simulink model "FOC"  (R2025a)
settings: Solver=VariableStepAuto  StartTime=0.0  StopTime=15  MaxStep=1e-4  RelTol=1e-3
undefined symbols (not defined in the file or in its folder): P
settings Model: Creator=20374  LastModifiedBy=20374

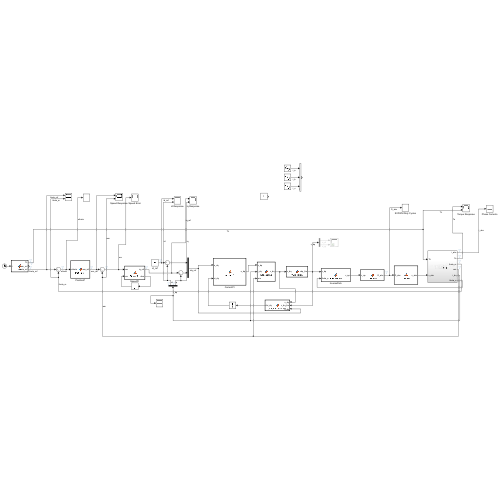
[thumbnail: Simulink's stored preview of the top-level diagram]
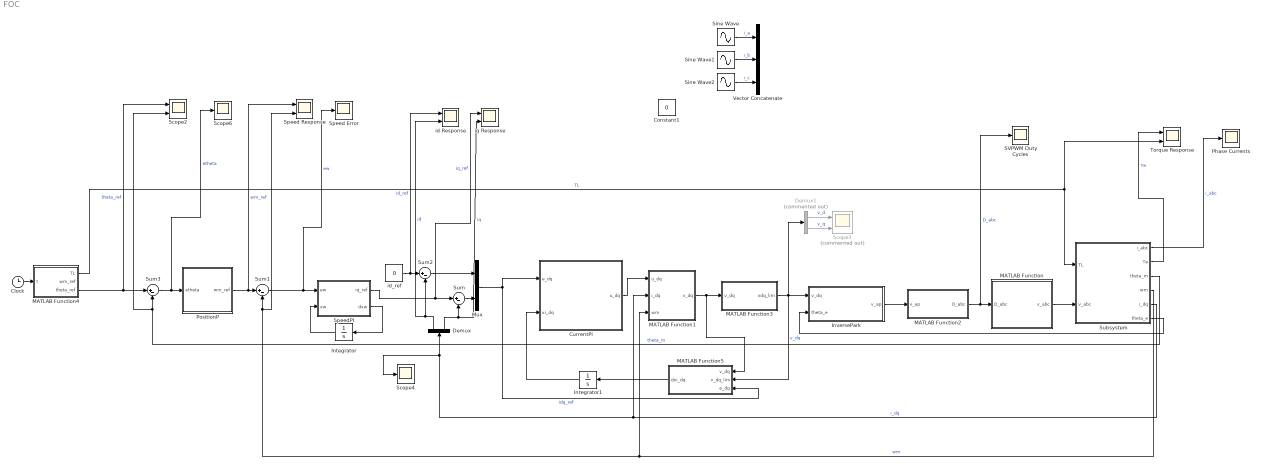
== system FOC ==
  Clock : Clock
  Constant1 : Constant  Value=0
  CurrentPI : MATLAB Function  TreatAsAtomicUnit=on
  Demux : Demux  Outputs=2
  Demux1 : Demux  Commented=on  Outputs=2
  Integrator : Integrator
  Integrator1 : Integrator
  InversePark : MATLAB Function  TreatAsAtomicUnit=on
  MATLAB Function : MATLAB Function  TreatAsAtomicUnit=on
  MATLAB Function1 : MATLAB Function  TreatAsAtomicUnit=on
  MATLAB Function2 : MATLAB Function  TreatAsAtomicUnit=on
  MATLAB Function3 : MATLAB Function  TreatAsAtomicUnit=on
  MATLAB Function4 : MATLAB Function  TreatAsAtomicUnit=on
  MATLAB Function5 : MATLAB Function  TreatAsAtomicUnit=on
  Mux : Mux  Inputs=2
  Phase Currents : Scope
      settings: DataLoggingVariableName=ScopeData9
  PositionP : MATLAB Function  TreatAsAtomicUnit=on
  SVPWM Duty Cycles : Scope
      settings: DataLoggingVariableName=ScopeData10
  Scope2 : Scope  NumInputPorts=2
      settings: ActiveDisplayYMinimum=-0.94255582944126726  ActiveDisplayYMaximum=16.800284873719775  DataLoggingVariableName=ScopeData2
  Scope3 : Scope  Commented=on  NumInputPorts=2
      settings: ActiveDisplayYMinimum=-185.69935334057905  ActiveDisplayYMaximum=341.38341103207864  DataLoggingVariableName=ScopeData3
  Scope4 : Scope
      settings: ActiveDisplayYMinimum=-1.2499772986958553  ActiveDisplayYMaximum=11.249795688208886  DataLoggingVariableName=ScopeData4
  Scope6 : Scope
      settings: ActiveDisplayYMinimum=-1.1047635267751033  ActiveDisplayYMaximum=7.10408082072833  DataLoggingVariableName=ScopeData7
  Sine Wave : Sin  Frequency=20*pi  SampleTime=0
  Sine Wave1 : Sin  Phase=2*pi/3  SampleTime=0
  Sine Wave2 : Sin  Phase=-2*pi/3  SampleTime=0
  Speed Error : Scope
      settings: ActiveDisplayYMinimum=-30.007135590035606  ActiveDisplayYMaximum=73.147296256443809  DataLoggingVariableName=ScopeData6
  Speed Response : Scope  NumInputPorts=2
      settings: ActiveDisplayYMinimum=-19.63649397524663  ActiveDisplayYMaximum=176.72844577721969  DataLoggingVariableName=ScopeData8
  SpeedPI : MATLAB Function  TreatAsAtomicUnit=on
  Subsystem : Subsystem
  Sum{,1..3} (4 alike) : Sum  Inputs=|+-
  Torque Response : Scope  NumInputPorts=2
      settings: DataLoggingVariableName=ScopeData5
  Vector Concatenate : Concatenate  NumInputs=3  Mode=Multidimensional array
  id Response : Scope  NumInputPorts=2
      settings: ActiveDisplayYMinimum=-27.477041816535841  ActiveDisplayYMaximum=247.29337634882265
  id_ref : Constant  Value=0
  iq Response : Scope  NumInputPorts=2
      settings: ActiveDisplayYMinimum=-6.574069056505973  ActiveDisplayYMaximum=11.841563228500664
  wires:
  Sine Wave/1 -> Vector Concatenate/1  "i_a"
  Sine Wave1/1 -> Vector Concatenate/2  "i_b"
  Sine Wave2/1 -> Vector Concatenate/3  "i_c"
  Integrator1/1 -> CurrentPI/2(xi_dq)
  CurrentPI/1(u_dq) -> MATLAB Function1/1(u_dq)
  Subsystem/6(theta_e) -> InversePark/2(theta_e)
  MATLAB Function/1(v_abc) -> Subsystem/2(v_abc)
  MATLAB Function2/1(D_abc) -> SVPWM Duty Cycles/1, MATLAB Function/1(D_abc)  "D_abc"
  InversePark/1(v_ap) -> MATLAB Function2/1(v_ap)
  Subsystem/5(i_dq) -> MATLAB Function1/2(i_dq), Scope4/1, Demux/1  "i_dq"
  Sum1/1 -> Speed Error/1, SpeedPI/1(ew)  "ew"
  Subsystem/4(wm) -> MATLAB Function1/3(wm), Speed Response/2, Sum1/2  "wm"
  MATLAB Function3/1(vdq_lim) -> Demux1/1, MATLAB Function5/2(v_dq_lim), InversePark/1(v_dq)  "v_dq"
  MATLAB Function1/1(v_dq) -> MATLAB Function5/1(v_dq), MATLAB Function3/1(v_dq)
  MATLAB Function4/1(TL) -> Torque Response/2, Subsystem/1(TL)  "TL"
  Clock/1 -> MATLAB Function4/1(t)
  Mux/1 -> CurrentPI/1(e_dq), MATLAB Function5/3(e_dq)  "idq_ref"
  Sum2/1 -> Mux/1
  Sum/1 -> Mux/2
  SpeedPI/1(iq_ref) -> iq Response/1, Sum/1  "iq_ref"
  id_ref/1 -> id Response/1, Sum2/1  "id_ref"
  Demux1/1 -> Scope3/1  "v_d"
  Demux1/2 -> Scope3/2  "v_q"
  Demux/1 -> Sum2/2, id Response/2  "id"
  Demux/2 -> Sum/2, iq Response/2  "iq"
  SpeedPI/2(dxw) -> Integrator/1
  Integrator/1 -> SpeedPI/2(xw)
  MATLAB Function5/1(dxi_dq) -> Integrator1/1
  Subsystem/3(theta_m) -> Scope2/2, Sum3/2  "theta_m"
  MATLAB Function4/3(theta_ref) -> Sum3/1, Scope2/1  "theta_ref"
  Sum3/1 -> Scope6/1, PositionP/1(etheta)  "etheta"
  Subsystem/2(Te) -> Torque Response/1  "Te"
  Subsystem/1(i_abc) -> Phase Currents/1  "i_abc"
  PositionP/1(wm_ref) -> Speed Response/1, Sum1/1  "wm_ref"

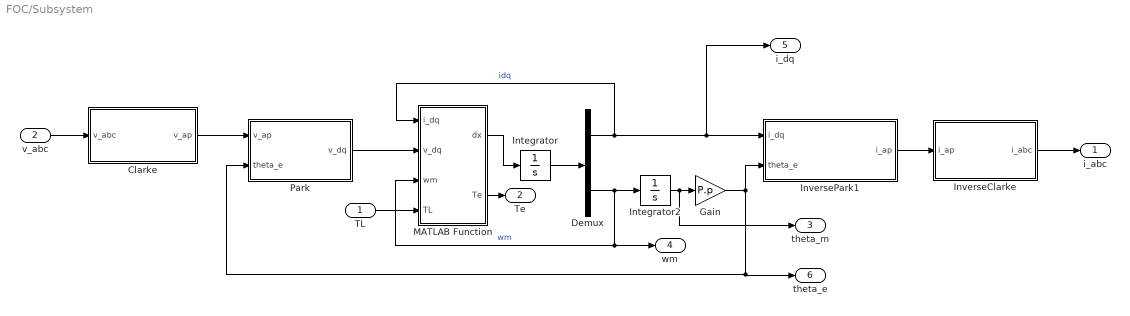
== system FOC/Subsystem ==
  TL : Inport
  v_abc : Inport  Port=2
  Clarke : MATLAB Function  TreatAsAtomicUnit=on
  Demux : Demux  Outputs=[2,1]
  Gain : Gain  Gain=P.p
  Integrator : Integrator  InitialCondition=[0;0;0]
  Integrator2 : Integrator
  InverseClarke : MATLAB Function  TreatAsAtomicUnit=on
  InversePark1 : MATLAB Function  TreatAsAtomicUnit=on
  MATLAB Function : MATLAB Function  TreatAsAtomicUnit=on
  Park : MATLAB Function  TreatAsAtomicUnit=on
  i_abc : Outport
  Te : Outport  Port=2
  theta_m : Outport  Port=3
  wm : Outport  Port=4
  i_dq : Outport  Port=5
  theta_e : Outport  Port=6
  wires:
  InversePark1/1(i_ap) -> InverseClarke/1(i_ap)
  Demux/2 -> wm/1, MATLAB Function/3(wm), Integrator2/1  "wm"
  Demux/1 -> i_dq/1, InversePark1/1(i_dq), MATLAB Function/1(i_dq)  "idq"
  Integrator2/1 -> theta_m/1, Gain/1
  Gain/1 -> theta_e/1, Park/2(theta_e), InversePark1/2(theta_e)
  TL/1 -> MATLAB Function/4(TL)
  Integrator/1 -> Demux/1
  InverseClarke/1(i_abc) -> i_abc/1
  MATLAB Function/1(dx) -> Integrator/1
  Clarke/1(v_ap) -> Park/1(v_ap)
  Park/1(v_dq) -> MATLAB Function/2(v_dq)
  v_abc/1 -> Clarke/1(v_abc)
  MATLAB Function/2(Te) -> Te/1

== matlab function FOC/MATLAB Function ==
  data: D_abc input; v_abc output; P parameter
function v_abc = Inverter(D_abc,P)

Da = D_abc(1);
Db = D_abc(2);
Dc = D_abc(3);

Vdc = P.Vdc;

va = Vdc/3 * (2*Da-Db-Dc);
vb = Vdc/3 * (2*Db-Da-Dc);
vc = Vdc/3 * (2*Dc-Da-Db);

v_abc = [va; vb; vc];

end

== matlab function FOC/MATLAB Function2 ==
  data: v_ap input; D_abc output; P parameter
function D_abc = SVPWM(v_ap,P)

v_alpha = v_ap(1);
v_beta  = v_ap(2);

Vdc = P.Vdc;
Ts  = P.Ts;

Da = 0;Db = 0;Dc = 0;
%% 1. Voltage vector magnitude and angle
v = sqrt(v_alpha^2 + v_beta^2);

theta = atan2(v_beta,v_alpha);

% Map theta to [0, 2*pi)
if theta < 0
    theta = theta + 2*pi;
end

sector = floor(theta/(pi/3)) + 1;

alpha = theta - (sector-1)*pi/3;

T1 = sqrt(3)*Ts*v/Vdc * sin(pi/3-alpha);
T2 = sqrt(3)*Ts*v/Vdc * sin(alpha);

T0 = Ts - T1 - T2;

%%
switch sector
    case 1
        Da = (T1 + T2 + T0/2)/Ts;
        Db = (T2 + T0/2)/Ts;
        Dc = (T0/2)/Ts;
    case 2
        Da = (T1 + T0/2)/Ts;
        Db = (T1 + T2 + T0/2)/Ts;
        Dc = (T0/2)/Ts;
    case 3
        Da = (T0/2)/Ts;
        Db = (T1 + T2 + T0/2)/Ts;
        Dc = (T2 + T0/2)/Ts;
    case 4
        Da = (T0/2)/Ts;
        Db = (T1 + T0/2)/Ts;
        Dc = (T1 + T2 + T0/2)/Ts;
    case 5
        Da = (T2 + T0/2)/Ts;
        Db = (T0/2)/Ts;
        Dc = (T1 + T2 + T0/2)/Ts;
    case 6
        Da = (T1 + T2 + T0/2)/Ts;
        Db = (T0/2)/Ts;
        Dc = (T1 + T0/2)/Ts;
end


D_abc = [Da;Db;Dc];

end

== matlab function FOC/MATLAB Function3 ==
  data: vdq_lim output; v_dq input; P parameter
function vdq_lim =  VLimitation(v_dq,P)

vd = v_dq(1);
vq = v_dq(2);

Vmax = P.Vdc/sqrt(3);

Vmag = sqrt(vd^2 + vq^2);

if Vmag > Vmax
    scale = Vmax/Vmag;
    vd = vd*scale;
    vq = vq*scale;
end

vdq_lim = [vd;vq];

== matlab function FOC/MATLAB Function4 ==
  data: TL output; wm_ref output; t input; theta_ref output
function [TL,wm_ref,theta_ref] = Ref(t)

%wm_ref
if t < 5
    wm_ref = 1000 * 2*pi/60;
else
    wm_ref = 1500 * 2*pi/60;
end

% theta_ref
if t < 5
    theta_ref = 2*pi;      % 1 revolution
else
    theta_ref = 4*pi;      % 2 revolutions
end

%TL
if t < 10
    TL = 0;
else
    TL = 2;
end

end

== matlab function FOC/MATLAB Function5 ==
  data: v_dq input; dxi_dq output; v_dq_lim input; e_dq input; P parameter
function dxi_dq = CurrentAntiWindup(v_dq,v_dq_lim,e_dq,P)

vd = v_dq(1);
vq = v_dq(2);
vd_lim = v_dq_lim(1);
vq_lim = v_dq_lim(2);
ed = e_dq(1);
eq = e_dq(2);

alpha_d = 1;       % adjustable between approximately 0.5 and 2
alpha_q = 1;

Kaw_d = 1/(alpha_d*P.Kpd);
Kaw_q = 1/(alpha_q*P.Kpq);

dxid = ed + Kaw_d*(vd_lim-vd);
dxiq = eq + Kaw_q*(vq_lim-vq);

dxi_dq = [dxid;
          dxiq];
end

== matlab function FOC/Subsystem/Park ==
  data: v_ap input; v_dq output; theta_e input
function v_dq = Park(v_ap, theta_e)

v_dq = [cos(theta_e)  , sin(theta_e);
        -sin(theta_e) , cos(theta_e)] * v_ap;

end

== matlab function FOC/Subsystem/Clarke ==
  data: v_abc input; v_ap output
function v_ap = Clarke(v_abc)

v_ap = 2/3 * [1 , -0.5      , -0.5;
              0 , sqrt(3)/2 , -sqrt(3)/2] * v_abc;

end

== matlab function FOC/Subsystem/InverseClarke ==
  data: i_ap input; i_abc output
function i_abc = InverseClarke(i_ap)

i_abc = [1 , 0;
         -0.5 , sqrt(3)/2;
         -0.5, -sqrt(3)/2] * i_ap;

end

== matlab function FOC/InversePark ==
  data: v_dq input; v_ap output; theta_e input
function v_ap = InversePark(v_dq,theta_e)

v_ap = [cos(theta_e) , -sin(theta_e);
        sin(theta_e) , cos(theta_e)] * v_dq;

end

== matlab function FOC/Subsystem/MATLAB Function ==
  data: i_dq input; dx output; v_dq input; wm input; TL input; P parameter; Te output
function [dx,Te] = PMSM(i_dq,v_dq,wm,TL, P)

id = i_dq(1);
iq = i_dq(2);
vd = v_dq(1);
vq = v_dq(2);

Rs = P.Rs;
Ld = P.Ld;
Lq = P.Lq;
phif = P.phif;
p = P.p;
B = P.B;
J = P.J;

we = p*wm;

did = (vd-Rs*id+we*Lq*iq)/Ld;
diq = (vq-Rs*iq-we*Ld*id-we*phif)/Lq;

Te = 3*p*(phif*iq+(Ld-Lq)*id*iq)/2;

dwm = (Te-TL-B*wm)/J;

dx = [did;diq;dwm];

end

== matlab function FOC/CurrentPI ==
  data: e_dq input size=[2 1]; xi_dq input size=[2 1]; P parameter; u_dq output size=[2 1]
function u_dq = CurrentPI(e_dq, xi_dq, P)

ed = e_dq(1);
eq = e_dq(2);

xid = xi_dq(1);
xiq = xi_dq(2);


ud = P.Kpd*ed + P.Kid*xid;
uq = P.Kpq*eq + P.Kiq*xiq;

u_dq = [ud;uq];

end

== matlab function FOC/SpeedPI ==
  settings: updateMethod=DISCRETE
  data: ew input; xw input; iq_ref output; P parameter; dxw output
function [iq_ref, dxw] = SpeedPI(ew, xw, P)
% ew  = wm_ref - wm
% xw  = speed integrator state
% dxw -> connect to speed Integrator input

Kp = P.Kpw;
Ki = P.Kiw;

Iq_max = 10;  % A

% Unsaturated PI output
iq0 = Kp*ew + Ki*xw;

% Current-reference saturation
iq_ref = min(max(iq0, -Iq_max), Iq_max);

% Back-calculation
% Corresponds to Tt = Kp/Ki
Kaw = 1/Kp;

dxw = ew + Kaw*(iq_ref - iq0);

end

== matlab function FOC/PositionP ==
  data: etheta input; wm_ref output; P parameter
function wm_ref = PositionP(etheta,P)

wm0 = P.Kpp * etheta;

% Speed reference limitation
wm_ref = min(max(wm0,-P.wm_max),P.wm_max);

end

== matlab function FOC/MATLAB Function1 ==
  data: u_dq input; i_dq input; wm input; v_dq output size=[2 1]; P parameter
function v_dq = Decoupling(u_dq,i_dq,wm,P)

ud = u_dq(1);
uq = u_dq(2);
id = i_dq(1);
iq = i_dq(2);

p = P.p;
Ld = P.Ld;
Lq = P.Lq;
phif = P.phif;

we = p*wm;

vd = ud-we*Lq*iq;
vq = uq+we*Ld*id+we*phif;

v_dq = [vd;vq];
end

== matlab function FOC/Subsystem/InversePark1 ==
  data: i_dq input; i_ap output; theta_e input
function i_ap = InversePark(i_dq,theta_e)

i_ap = [cos(theta_e) , -sin(theta_e);
        sin(theta_e) , cos(theta_e)] * i_dq;

end
